simulink model "iso_calc_temp_ver3"  (Simulink 8.7)
settings: Solver=VariableStepAuto  SolverMode=SingleTasking  StartTime=0.0  StopTime=inf  RelTol=1e-6
values from neighbouring files (symbols this model uses):
  C = 1    [DataLoop.m]    (also in run_iso_calc.m; testLoop.m = 1.2)
  t_current = 0    [DataLoop.m]    (also in run_iso_calc.m = (0:t_process:tf)'; testLoop.m)
  Tr = 1    [DataLoop.m]    (also in run_iso_calc.m = 0; testLoop.m = 0.38)
  Ts = 1    [DataLoop.m]    (also in run_iso_calc.m = 0; testLoop.m = 0.5)
  Vs = 1    [DataLoop.m]    (also in run_iso_calc.m = -Vh; testLoop.m = 0)
  Zd = 1    [DataLoop.m]    (also in run_iso_calc.m = 0.05; testLoop.m = 0.02)
  Zr = 1    [DataLoop.m]    (also in run_iso_calc.m = 0; testLoop.m = 0)
libraries: simulink x1
settings Model: Creator=laiy  LastModifiedBy=jake
settings DataIOCC: LimitDataPoints=off  SaveFormat=Dataset  ReturnWorkspaceOutputs=on
settings DebuggingCC: UnderspecifiedInitializationDetection=Simplified  MergeDetectMultiDrivingBlocksExec=error  SFUnexpectedBacktrackingDiag=error  SFNoUnconditionalDefaultTransitionDiag=error
settings HardwareCC: ProdBitPerPointer=64  ProdLargestAtomicFloat=Float  ProdIntDivRoundTo=Zero  ProdEndianess=LittleEndian  ProdWordSize=64  ProdHWDeviceType=Intel->x86-64 (Windows64)
settings ModelReferenceCC: PropagateSignalLabelsOutOfModel=on
settings SFSimCC: SimUseLocalCustomCode=on
settings RTWCC: RTWUseLocalCustomCode=on
settings GRTTargetCC: TargetLangStandard=C99 (ISO)
settings ConfigComp: CovMetricSettings=dwe  CovHtmlReporting=off  CovSaveCumulativeToWorkspaceVar=off  CovSaveSingleToWorkspaceVar=off  CovModelRefEnable=off  CovExternalEMLEnable=on

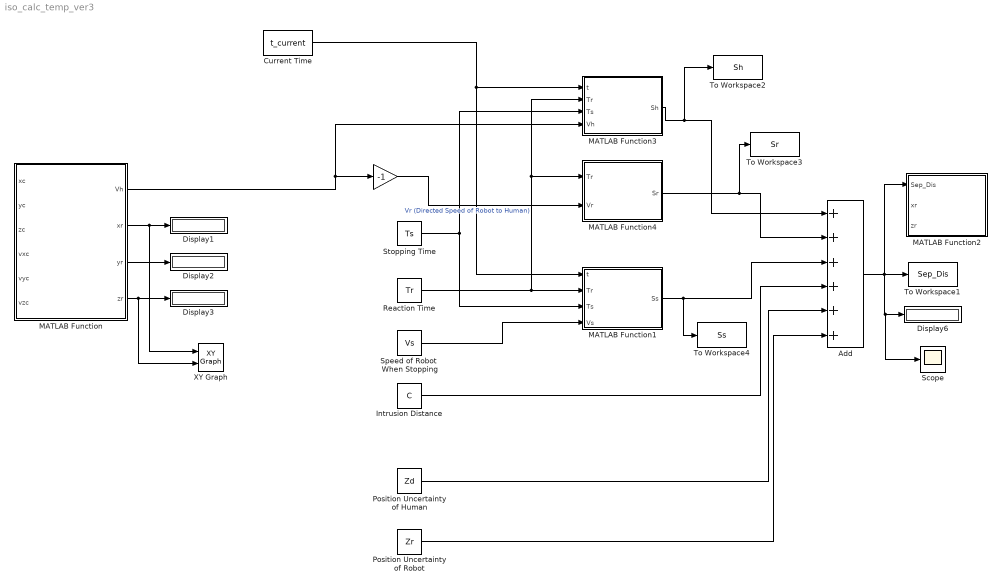
== system iso_calc_temp_ver3 ==
  " " : Gain  Gain=-1
  Add : Sum  Inputs=++++++
  Current Time : Constant  Value=t_current
  Display{1..3,6} (4 alike) : Display
  Intrusion Distance : Constant  Value=C
  MATLAB Function : MATLAB Function  TreatAsAtomicUnit=on
  MATLAB Function1 : MATLAB Function  TreatAsAtomicUnit=on
  MATLAB Function2 : MATLAB Function  TreatAsAtomicUnit=on
  MATLAB Function3 : MATLAB Function  TreatAsAtomicUnit=on
  MATLAB Function4 : MATLAB Function  TreatAsAtomicUnit=on
  Position Uncertainty of Human : Constant  Value=Zd
  Position Uncertainty of Robot : Constant  Value=Zr
  Reaction Time : Constant  Value=Tr
  Scope : Scope
  Speed of Robot  When Stopping : Constant  Value=Vs
  Stopping Time : Constant  Value=Ts
  To Workspace1 : ToWorkspace  VariableName=Sep_Dis  SampleTime=-1
  To Workspace2 : ToWorkspace  VariableName=Sh  SampleTime=-1
  To Workspace3 : ToWorkspace  VariableName=Sr  SampleTime=-1
  To Workspace4 : ToWorkspace  VariableName=Ss  SampleTime=-1
  XY Graph : simulink/Sinks/XY Graph  xmin=-10  xmax=10  ymin=10  ymax=10  st=-1
  wires:
  MATLAB Function1/1(Ss) -> To Workspace4/1, Add/3
  MATLAB Function3/1(Sh) -> To Workspace2/1, Add/1
  MATLAB Function4/1(Sr) -> To Workspace3/1, Add/2
  Intrusion Distance/1 -> Add/4
  Position Uncertainty of Human/1 -> Add/5
  Position Uncertainty of Robot/1 -> Add/6
  Reaction Time/1 -> MATLAB Function1/2(Tr), MATLAB Function4/1(Tr), MATLAB Function3/2(Tr)
  Stopping Time/1 -> MATLAB Function3/3(Ts), MATLAB Function1/3(Ts)
  " "/1 -> MATLAB Function4/2(Vr)  "Vr (Directed Speed of Robot to Human)"
  Current Time/1 -> MATLAB Function1/1(t), MATLAB Function3/1(t)
  Speed of Robot  When Stopping/1 -> MATLAB Function1/4(Vs)
  Add/1 -> MATLAB Function2/1(Sep_Dis), Scope/1, Display6/1, To Workspace1/1
  MATLAB Function/1(Vh) -> MATLAB Function3/4(Vh), " "/1
  MATLAB Function/2(xr) -> XY Graph/1, Display1/1
  MATLAB Function/3(yr) -> Display2/1
  MATLAB Function/4(zr) -> XY Graph/2, Display3/1

== matlab function MATLAB Function4 ==
  data: Tr input double; Vr input double; Sr output double
function Sr = fcn(Tr, Vr)

% separation distance due to robot motion
% Vr is assumed to reduces the separation distance the most

Sr = Tr * Vr;

== matlab function MATLAB Function3 ==
  data: t input double; Sh output double; Tr input double; Ts input double; Vh input double
function Sh = fcn(t, Tr, Ts, Vh)

% separation distance due to operator's change in location

t_int = t:0.001:t+Tr+Ts;
v = zeros(length(t_int),1) + Vh;

Sh = trapz(t_int,v);

== matlab function MATLAB Function1 ==
  data: t input double; Tr input double; Ss output double; Ts input double; Vs input double
function Ss = fcn(t, Tr, Ts, Vs)

% separation distance due to robot stopping

t_int = t+Tr:0.001:t+Tr+Ts;
v = zeros(length(t_int),1) + Vs;

Ss = trapz(t_int,v);

== matlab function MATLAB Function2 ==
  data: Sep_Dis input double; xr input double; zr input double
function display(Sep_Dis, xr,zr)

fprintf(1, 'Separation Distance: %f\n', Sep_Dis(1,1));

fileID = fopen('output.txt','w');
fprintf(fileID,'%f\n',Sep_Dis);
fclose(fileID);


f = figure(1);
title('Separation Distance');
plot(xr*5,zr*5,'o','MarkerSize', 3, 'MarkerFaceColor', 'black');
hold on;
plot(0,0,'o','MarkerSize',1, 'LineWidth', 3, 'Color', 'Red','MarkerSize', int8(abs(Sep_Dis)*100));
hold off;
xlim([-5,5]);
ylim([-5,5]);

if sqrt(xr^2 + zr^2) <= Sep_Dis
    fprintf(1,'DANGER');
end

== matlab function MATLAB Function ==
  data: xc input double; Vh output double; yc input double; zc input double; vxc input double; vyc input double; vzc input double; xr output double; yr output double; zr output double
function [Vh,xr,yr,zr] = find_Vh(xc,yc,zc,vxc,vyc,vzc)

[xr,yr,zr,vxr,vyr,vzr] = trans_cam_rob(xc,yc,zc,vxc,vyc,vzc);

Vh = sqrt(vxr^2 + vzr^2);
